simulink model "hexa_flat"  (R2023a)
settings: Solver=ode4  StartTime=0.0  StopTime=tf  FixedStep=0.01  RelTol=1e-3
model workspace (MAT data in the model file):
  tf = Simulink.Parameter
  tf.Value = 60
  tf.DataType = 'auto'
  tf.Complexity = 'real'
  tf.Dimensions = [1 1]
  tray2 = [0  2  2  -2  -2  0; 0  0  -2  -2  2  0; 0  5  2.5  5  2.5  0; 0  0  0  0  0  0; 0  0  0  0  0  0; 0  0  0  0  0  0]
libraries: robotcorelib x1
settings Model: Creator=adan  LastModifiedBy=Adan Daniel
settings OptimizationCC: ReuseModelBlockBuffer=off

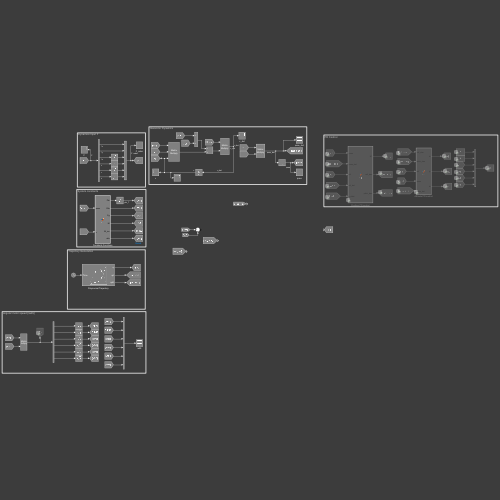
[thumbnail: Simulink's stored preview of the top-level diagram]
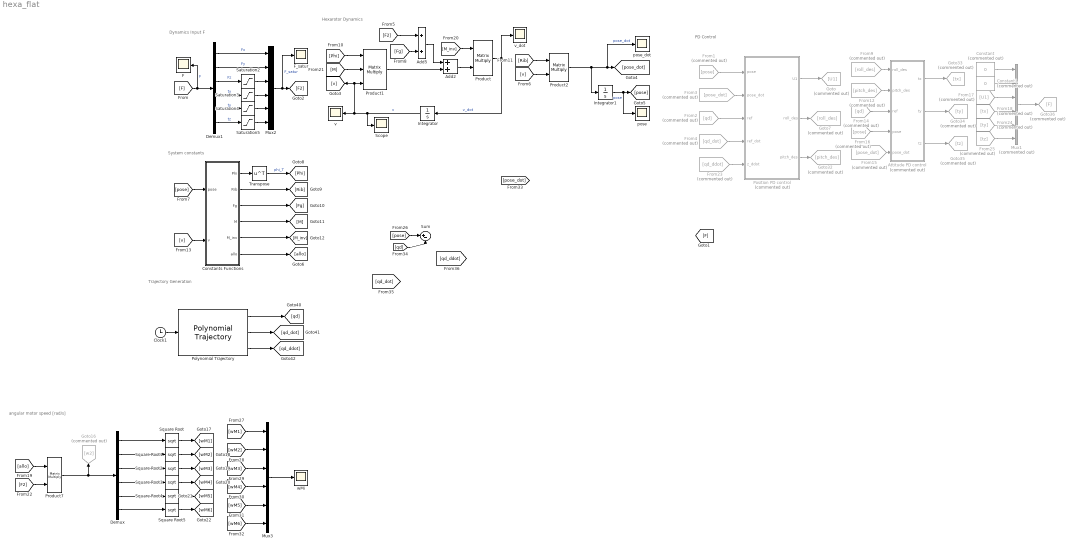
== system hexa_flat ==
  note: angular motor speed [rad/s]
  note: System constants
  note: PD Control
  note: Hexarotor Dynamics
  note: Dynamics Input F
  note: Trajectory Generation
  Add2 : Sum
  Add5 : Sum
  Attitude PD control : MATLAB Function  Commented=on  TreatAsAtomicUnit=on
  Clock1 : Clock
  Constant : Constant  Commented=on  Value=0
  Constant1 : Constant  Commented=on  Value=0
  Constants Functions : MATLAB Function  TreatAsAtomicUnit=on
  Demux : Demux  Outputs=6
  Demux1 : Demux  Outputs=6
  F : Scope
  F_satur : Scope
  From1 : From  Commented=on  GotoTag=pose
  From12 : From  Commented=on  GotoTag=pitch_des
  From14 : From  Commented=on  GotoTag=qd
  From15 : From  Commented=on  GotoTag=pose_dot
  From16 : From  Commented=on  GotoTag=pose
  From17 : From  Commented=on  GotoTag=U1
  From18 : From  Commented=on  GotoTag=tx
  From2 : From  Commented=on  GotoTag=qd
  From23 : From  Commented=on  GotoTag=qd_ddot
  From24 : From  Commented=on  GotoTag=ty
  From25 : From  Commented=on  GotoTag=tz
  From3 : From  Commented=on  GotoTag=pose_dot
  From4 : From  Commented=on  GotoTag=qd_dot
  From9 : From  Commented=on  GotoTag=roll_des
  Goto : Goto  Commented=on  GotoTag=U1
  Goto16 : Goto  Commented=on  GotoTag=w2
  Goto32 : Goto  Commented=on  GotoTag=pitch_des
  Goto33 : Goto  Commented=on  GotoTag=tx
  Goto34 : Goto  Commented=on  GotoTag=ty
  Goto35 : Goto  Commented=on  GotoTag=tz
  Goto36 : Goto  Commented=on  GotoTag=F
  Goto7 : Goto  Commented=on  GotoTag=roll_des
  Integrator : Integrator  InitialCondition=[0; 0; 0; 0; 0; 0]
  Integrator1 : Integrator  InitialCondition=[0; 0; 0; 0; 0; 0]
  Mux1 : Mux  Commented=on  Inputs=6
  Mux2 : Mux  Inputs=6
  Mux3 : Mux  Inputs=6
  Polynomial Trajectory : robotcorelib/Polynomial Trajectory  WaypointSource=Internal  Waypoints=tray2  TimePoints=[ 0, 12, 24, 35, 48, tf ]  TimeInterval=[ 1, 4 ]  Method=Cubic Polynomial  ParameterSource=Internal  VelocityBoundaryCondition=zeros( 6, 6 )  AccelerationBoundaryCondition=zeros( 2, 5 )  SimulateUsing=Interpreted execution
  Position PD control : MATLAB Function  Commented=on  TreatAsAtomicUnit=on
  Product : Product  Multiplication=Matrix(*)
  Product1 : Product  Inputs=3  Multiplication=Matrix(*)
  Product2 : Product  Multiplication=Matrix(*)
  Product7 : Product  Multiplication=Matrix(*)
  Saturation2 : Saturate  UpperLimit=5.8*6  LowerLimit=0
  Saturation3 : Saturate
  Saturation4 : Saturate
  Saturation5 : Saturate
  Scope : Scope
  Square Root{,1..5} (6 alike) : Sqrt
  Sum : Sum  Inputs=|+-
  Transpose : Math  Operator=transpose
  pose : Scope
  pose_dot : Scope
  v : Scope
  v_dot : Scope
  wMi : Scope
  wires:
  Saturation4/1 -> Mux2/5
  Saturation3/1 -> Mux2/4
  Demux1/6 -> Saturation5/1  "tz"
  Demux1/3 -> Saturation2/1  "Fz"
  [F] -> F/1, Demux1/1  "F"
  Saturation5/1 -> Mux2/6
  Demux1/2 -> Mux2/2  "Fy"
  Demux1/1 -> Mux2/1  "Fx"
  Demux1/5 -> Saturation4/1  "ty"
  Demux1/4 -> Saturation3/1  "tx"
  Saturation2/1 -> Mux2/3
  Mux2/1 -> F_satur/1, [F2]  "F_satur"
  [M] -> Product1/2
  [v] -> Product2/2
  [M_inv] -> Product/1
  Add2/1 -> Product/2
  Product/1 -> v_dot/1, Integrator/1  "v_dot"
  [Rib] -> Product2/1
  Product2/1 -> Integrator1/1, pose_dot/1, [pose_dot]  "pose_dot"
  [Phi] -> Product1/1
  Product1/1 -> Add2/2
  Integrator1/1 -> pose/1, [pose]  "pose"
  Integrator/1 -> Scope/1, v/1, [v], Product1/3  "v"
  [Fg] -> Add5/2
  Add5/1 -> Add2/1
  [F2] -> Add5/1
  From18/1 -> Mux1/4
  Constant1/1 -> Mux1/2
  From16/1 -> Attitude PD control/4(pose)
  Mux1/1 -> Goto36/1
  From15/1 -> Attitude PD control/5(pose_dot)
  Attitude PD control/1(tx) -> Goto33/1
  Constant/1 -> Mux1/1
  From12/1 -> Attitude PD control/2(pitch_des)
  Attitude PD control/2(ty) -> Goto34/1
  Position PD control/1(U1) -> Goto/1
  From1/1 -> Position PD control/1(pose)
  Position PD control/2(roll_des) -> Goto7/1
  Attitude PD control/3(tz) -> Goto35/1
  From17/1 -> Mux1/3
  Position PD control/3(pitch_des) -> Goto32/1
  From9/1 -> Attitude PD control/1(roll_des)
  From4/1 -> Position PD control/4(ref_dot)
  From24/1 -> Mux1/5
  From14/1 -> Attitude PD control/3(ref)
  From3/1 -> Position PD control/2(pose_dot)
  From2/1 -> Position PD control/3(ref)
  From25/1 -> Mux1/6
  Constants Functions/1(Phi) -> Transpose/1
  Constants Functions/3(Fg) -> [Fg]
  Constants Functions/2(Rib) -> [Rib]
  Transpose/1 -> [Phi]  "phi_T"
  Constants Functions/5(M_inv) -> [M_inv]
  Constants Functions/4(M) -> [M]
  Constants Functions/6(allo) -> [allo]
  [v] -> Constants Functions/2(v)
  [pose] -> Constants Functions/1(pose)
  [wM3] -> Mux3/3
  [allo] -> Product7/1
  [wM6] -> Mux3/6
  [wM2] -> Mux3/2
  Demux/2 -> Square Root1/1
  Product7/1 -> Demux/1, Goto16/1
  Demux/6 -> Square Root5/1
  Demux/5 -> Square Root4/1
  [wM4] -> Mux3/4
  Mux3/1 -> wMi/1
  Square Root2/1 -> [wM3]
  Demux/4 -> Square Root3/1
  Demux/1 -> Square Root/1
  [wM1] -> Mux3/1
  [F2] -> Product7/2
  Square Root1/1 -> [wM2]
  [wM5] -> Mux3/5
  Square Root4/1 -> [wM5]
  Demux/3 -> Square Root2/1
  Square Root5/1 -> [wM6]
  Square Root3/1 -> [wM4]
  Square Root/1 -> [wM1]
  Polynomial Trajectory/1 -> [qd]
  Clock1/1 -> Polynomial Trajectory/1
  Polynomial Trajectory/2 -> [qd_dot]
  Polynomial Trajectory/3 -> [qd_ddot]
  From23/1 -> Position PD control/5(z_ddot)
  [pose] -> Sum/1
  [qd] -> Sum/2

== matlab function hexa_flat/Constants Functions ==
  data: Phi output; Rib output; Fg output; pose input; M output; M_inv output; v input; allo output
function [Phi, Rib, Fg, M, M_inv, allo]   = fcn(pose, v)

%% System constants
m = 1.525; %5 mass 2.2 kg
l = 0.27; % m
g = 9.81; % gravity
Jxx =  0.0411; % kg m²
Jyy = 0.0478; % kg m²
Jzz = 0.0599; % kg m²
kT = 3.4e-5;
kQ = 3.4e-6;
%% Phi vector 6d

uu = v(1);
vv = v(2);
ww = v(3);
pp = v(4);
qq = v(5);
rr = v(6);


Phi = [0, -rr, qq, 0, -ww, vv;
        rr, 0, -pp , ww, 0, -uu;
        -qq, pp, 0,  -vv, uu, 0;
        0, 0, 0, 0, -rr, qq; 
        0, 0, 0, rr, 0, -pp;
        0, 0, 0, -qq, pp, 0];
%% Fg and Rib calculation

roll = pose(4);
pitch = pose(5);
yaw = pose(6);


Rib = [cos(yaw)*cos(pitch), -cos(roll)*sin(yaw) + cos(yaw)*sin(roll)*sin(pitch), sin(roll)*sin(yaw) + cos(roll)*cos(yaw)*sin(pitch), 0, 0, 0;
       cos(pitch)*sin(yaw), cos(roll)*cos(yaw) + sin(yaw)*sin(pitch)*sin(roll), -cos(yaw)*sin(roll) + sin(yaw)*sin(pitch)*cos(roll), 0, 0, 0;
       -sin(pitch), cos(pitch)*sin(roll), cos(pitch)*cos(roll), 0, 0, 0;
       0, 0, 0, 1, sin(roll)*tan(pitch), cos(roll)*tan(pitch);
       0, 0, 0, 0, cos(roll), -sin(roll);
       0, 0, 0, 0, sin(roll)/cos(pitch), cos(roll)/cos(pitch)];

Fg = [m*g*sin(pitch);
      -m*g*cos(pitch)*sin(roll);
      -m*g*cos(pitch)*cos(roll);
      0;
      0;
      0];

%% M matrix

M = [m, 0, 0, 0, 0, 0;
    0, m, 0, 0, 0, 0;
    0, 0, m, 0, 0, 0;
    0, 0, 0, Jxx, 0, 0;
    0, 0, 0, 0, Jyy, 0;
    0, 0, 0, 0, 0, Jzz];

M_inv = inv(M);

%% Allocation matrix

allo = [0, 0, 0, 0, 0, 0;
        0, 0, 0, 0, 0, 0;
        kT, kT, kT, kT, kT, kT;
        -kT*l, kT*l, kT*l/2, -kT*l/2, -kT*l/2, kT*l/2;
        0, 0, -sqrt(3)*kT*l/2, sqrt(3)*kT*l/2, -sqrt(3)*kT*l/2, sqrt(3)*kT*l/2;
        kQ, -kQ, kQ, -kQ, -kQ, kQ,];

allo = pinv(allo);

== matlab function hexa_flat/Position PD control ==
  data: pose input; U1 output; pose_dot input; ref input; ref_dot input; z_ddot input; roll_des output; pitch_des output
function [U1, roll_des, pitch_des] = fcn(pose, pose_dot, ref, ref_dot, z_ddot)

m = 2.0;
g = 9.81;
z_ddot = 0;

%% Determine u_uax_z

z_real = pose(3);
z_real_dot = pose_dot(3);
z_d = ref(3);
% z_d_dot = ref_dot(3);

error_z = z_d - z_real;
error_z_dot = - z_real_dot;

kp_z = 7;
kd_z = 5;

u_aux_z = kp_z*error_z + kd_z*error_z_dot; 

%% Determine u_uax_x andd u_uax_y

x_real = pose(1);
x_real_dot = pose_dot(1);
x_d = ref(1);
% x_d_dot = ref_dot(1);

error_x = x_d - x_real;
error_x_dot = - x_real_dot;

kp_x = 1.5;
kd_x = 2.5;

u_uax_x = kp_x*error_x + kd_x*error_x_dot;
% u_uax_x = - u_uax_x;

y_real = pose(2);
y_real_dot = pose_dot(2);
y_d = ref(2);
% y_d_dot = ref_dot(2);

error_y = y_d - y_real;
error_y_dot =  - y_real_dot;

kp_y = 1.5;
kd_y = 2.5;

u_uax_y = kp_y*error_y + kd_y*error_y_dot;
% u_uax_y = - u_uax_y;

%% Roll and Pitch

roll = pose(4);
pitch = pose(5);
yaw = ref(6);

%% Calculate thrust U1

U1 = (m/(cos(roll)*cos(pitch)))*(z_ddot - g + u_aux_z);

%% Calculate roll and pitch desired

% roll_des = asin(((m/U1)*u_uax_x*sin(yaw)) - ((m/U1)*u_uax_y*cos(yaw)));
roll_des_calculation = ((m/U1)*u_uax_x*sin(yaw)) - ((m/U1)*u_uax_y*cos(yaw));


if roll_des_calculation > 1
    roll_des_calculation = 1;
elseif roll_des_calculation < -1
    roll_des_calculation = -1;
end
roll_des = asin(roll_des_calculation);

pitch_des_calculation = (((m/U1)*u_uax_x) - (sin(roll_des)*sin(yaw)))/(cos(roll_des)*cos(yaw));
if (pitch_des_calculation > 1)
    pitch_des_calculation = 1;
elseif (pitch_des_calculation < -1)
    pitch_des_calculation = -1;
end

pitch_des = asin(pitch_des_calculation);

== matlab function hexa_flat/Attitude PD control ==
  data: roll_des input; tx output; pitch_des input; ref input; pose input; pose_dot input; ty output; tz output
function [tx, ty, tz]= fcn(roll_des, pitch_des, ref, pose, pose_dot)

%% u_uax_roll and u_uax_pitch



roll_real = pose(4);
roll_real_dot = pose_dot(4);
roll_d = roll_des;

error_roll = roll_d - roll_real;
error_roll_dot = - roll_real_dot;

kp_roll = 25;
kd_roll = 7.5;
u_uax_roll = kp_roll*error_roll + kd_roll*error_roll_dot;
tx = Jxx*u_uax_roll - (Jyy - Jzz)*pose_dot(4)*pose_dot(5);

pitch_real = pose(5);
pitch_real_dot = pose_dot(5);
pitch_d = pitch_des;

error_pitch= pitch_d - pitch_real;
error_pitch_dot = - pitch_real_dot;

kp_pitch = 20;
kd_pitch = 10;

u_uax_pitch = kp_pitch*error_pitch + kd_pitch*error_pitch_dot;
ty = Jyy*u_uax_pitch - (Jzz - Jxx)*pose_dot(3)*pose_dot(5);


%% u_uax_yaw

yaw_real = pose(6);
yaw_real_dot = pose_dot(6);
yaw_d = ref(6);

error_yaw = yaw_d - yaw_real;
error_yaw_dot = - yaw_real_dot;

kp_yaw = 1;
kd_yaw = 1;

u_uax_yaw = kp_yaw*error_yaw + kd_yaw*error_yaw_dot;
tz = Jzz*u_uax_yaw - (Jxx - Jyy)*pose_dot(3)*pose_dot(4);
